simulink library "MBDS_Applications"  (R2018b)
settings: Solver=ode45  StartTime=0.0  StopTime=10.0  RelTol=1e-3
undefined symbols (not defined in the file or in its folder): Ts
libraries: KIBES_Signal x297, simulink x7
(part 3 of 6)

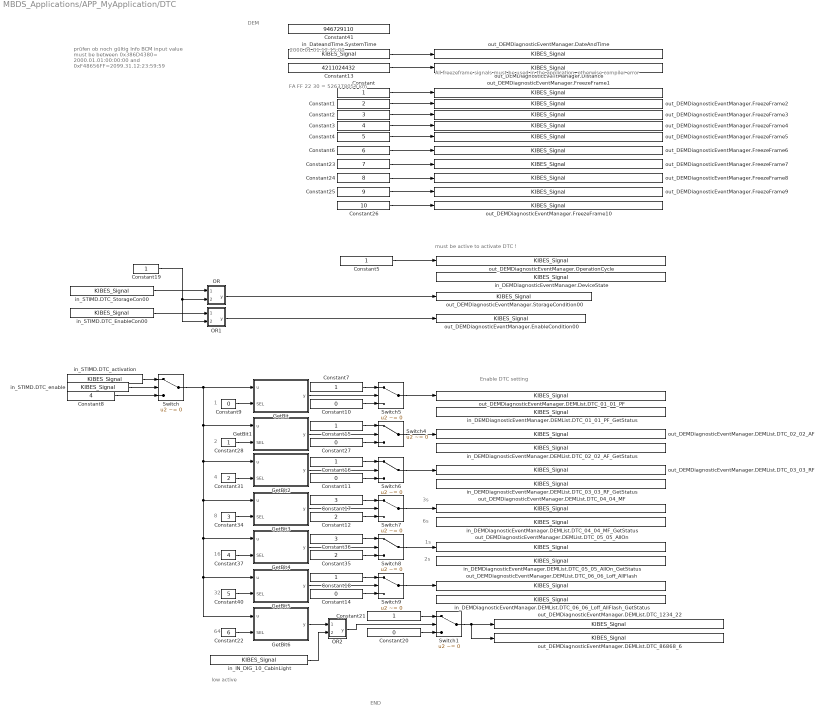
== system MBDS_Applications/APP_MyApplication/DTC ==
  note: 64
  note: FA FF 22 30 = 526378054 km
  note: 2000.01.01:12:15:00
  note: DEM
  note: prüfen ob noch gültig Info BCM
      | input value must be between
      | 0x386D4380= 2000.01.01:00:00:00 and
      | 0xF48656FF=2099.31.12:23:59:59
  note: must be active to activate DTC !
  note: Enable DTC setting
  note: END
  note: 1
  note: 2
  note: 4
  note: 8
  note: 16
  note: 32
  note: 3s
  note: 6s
  note: 1s
  note: 2s
  note: All freezeframe signals must be used in the application, otherwise compiler error
  note: low active
  Constant : Constant  InitFcn=|  OutDataTypeStr=uint16
      | if(exist('MBDS_BlockCallback', 'file'))
      |    MBDS_BlockCallback('Update', gcb);  
      | end
  Constant1 : Constant  InitFcn=|  Value=2  OutDataTypeStr=uint16
      | if(exist('MBDS_BlockCallback', 'file'))
      |    MBDS_BlockCallback('Update', gcb);  
      | end
  Constant10 : Constant  InitFcn=|  Value=0  OutDataTypeStr=uint8
      | if(exist('MBDS_BlockCallback', 'file'))
      |    MBDS_BlockCallback('Update', gcb);  
      | end
  Constant11 : Constant  InitFcn=|  Value=0  OutDataTypeStr=uint8
      | if(exist('MBDS_BlockCallback', 'file'))
      |    MBDS_BlockCallback('Update', gcb);  
      | end
  Constant12 : Constant  InitFcn=|  Value=2  OutDataTypeStr=uint8
      | if(exist('MBDS_BlockCallback', 'file'))
      |    MBDS_BlockCallback('Update', gcb);  
      | end
  Constant13 : Constant  InitFcn=|  Value=4211024432  OutDataTypeStr=uint32
      | if(exist('MBDS_BlockCallback', 'file'))
      |    MBDS_BlockCallback('Update', gcb);  
      | end
  Constant14 : Constant  InitFcn=|  Value=0  OutDataTypeStr=uint8
      | if(exist('MBDS_BlockCallback', 'file'))
      |    MBDS_BlockCallback('Update', gcb);  
      | end
  Constant15 : Constant  InitFcn=|  OutDataTypeStr=uint8
      | if(exist('MBDS_BlockCallback', 'file'))
      |    MBDS_BlockCallback('Update', gcb);  
      | end
  Constant16 : Constant  InitFcn=|  OutDataTypeStr=uint8
      | if(exist('MBDS_BlockCallback', 'file'))
      |    MBDS_BlockCallback('Update', gcb);  
      | end
  Constant17 : Constant  InitFcn=|  Value=3  OutDataTypeStr=uint8
      | if(exist('MBDS_BlockCallback', 'file'))
      |    MBDS_BlockCallback('Update', gcb);  
      | end
  Constant18 : Constant  InitFcn=|  OutDataTypeStr=uint8
      | if(exist('MBDS_BlockCallback', 'file'))
      |    MBDS_BlockCallback('Update', gcb);  
      | end
  Constant19 : Constant  InitFcn=|  OutDataTypeStr=boolean
      | if(exist('MBDS_BlockCallback', 'file'))
      |    MBDS_BlockCallback('Update', gcb);  
      | end
  Constant2 : Constant  InitFcn=|  Value=3  OutDataTypeStr=uint16
      | if(exist('MBDS_BlockCallback', 'file'))
      |    MBDS_BlockCallback('Update', gcb);  
      | end
  Constant20 : Constant  InitFcn=|  Value=0  OutDataTypeStr=uint8
      | if(exist('MBDS_BlockCallback', 'file'))
      |    MBDS_BlockCallback('Update', gcb);  
      | end
  Constant21 : Constant  InitFcn=|  OutDataTypeStr=uint8
      | if(exist('MBDS_BlockCallback', 'file'))
      |    MBDS_BlockCallback('Update', gcb);  
      | end
  Constant22 : Constant  InitFcn=|  Value=6  OutDataTypeStr=uint8
      | if(exist('MBDS_BlockCallback', 'file'))
      |    MBDS_BlockCallback('Update', gcb);  
      | end
  Constant23 : Constant  InitFcn=|  Value=7  OutDataTypeStr=uint16
      | if(exist('MBDS_BlockCallback', 'file'))
      |    MBDS_BlockCallback('Update', gcb);  
      | end
  Constant24 : Constant  InitFcn=|  Value=8  OutDataTypeStr=uint16
      | if(exist('MBDS_BlockCallback', 'file'))
      |    MBDS_BlockCallback('Update', gcb);  
      | end
  Constant25 : Constant  InitFcn=|  Value=9  OutDataTypeStr=uint16
      | if(exist('MBDS_BlockCallback', 'file'))
      |    MBDS_BlockCallback('Update', gcb);  
      | end
  Constant26 : Constant  InitFcn=|  Value=10  OutDataTypeStr=uint16
      | if(exist('MBDS_BlockCallback', 'file'))
      |    MBDS_BlockCallback('Update', gcb);  
      | end
  Constant27 : Constant  InitFcn=|  Value=0  OutDataTypeStr=uint8
      | if(exist('MBDS_BlockCallback', 'file'))
      |    MBDS_BlockCallback('Update', gcb);  
      | end
  Constant28 : Constant  InitFcn=|  OutDataTypeStr=uint8
      | if(exist('MBDS_BlockCallback', 'file'))
      |    MBDS_BlockCallback('Update', gcb);  
      | end
  Constant3 : Constant  InitFcn=|  Value=4  OutDataTypeStr=uint16
      | if(exist('MBDS_BlockCallback', 'file'))
      |    MBDS_BlockCallback('Update', gcb);  
      | end
  Constant31 : Constant  InitFcn=|  Value=2  OutDataTypeStr=uint8
      | if(exist('MBDS_BlockCallback', 'file'))
      |    MBDS_BlockCallback('Update', gcb);  
      | end
  Constant34 : Constant  InitFcn=|  Value=3  OutDataTypeStr=uint8
      | if(exist('MBDS_BlockCallback', 'file'))
      |    MBDS_BlockCallback('Update', gcb);  
      | end
  Constant35 : Constant  InitFcn=|  Value=2  OutDataTypeStr=uint8
      | if(exist('MBDS_BlockCallback', 'file'))
      |    MBDS_BlockCallback('Update', gcb);  
      | end
  Constant36 : Constant  InitFcn=|  Value=3  OutDataTypeStr=uint8
      | if(exist('MBDS_BlockCallback', 'file'))
      |    MBDS_BlockCallback('Update', gcb);  
      | end
  Constant37 : Constant  InitFcn=|  Value=4  OutDataTypeStr=uint8
      | if(exist('MBDS_BlockCallback', 'file'))
      |    MBDS_BlockCallback('Update', gcb);  
      | end
  Constant4 : Constant  InitFcn=|  Value=5  OutDataTypeStr=uint16
      | if(exist('MBDS_BlockCallback', 'file'))
      |    MBDS_BlockCallback('Update', gcb);  
      | end
  Constant40 : Constant  InitFcn=|  Value=5  OutDataTypeStr=uint8
      | if(exist('MBDS_BlockCallback', 'file'))
      |    MBDS_BlockCallback('Update', gcb);  
      | end
  Constant41 : Constant  InitFcn=|  Value=946729110  OutDataTypeStr=uint32
      | if(exist('MBDS_BlockCallback', 'file'))
      |    MBDS_BlockCallback('Update', gcb);  
      | end
  Constant5 : Constant  InitFcn=|  OutDataTypeStr=boolean
      | if(exist('MBDS_BlockCallback', 'file'))
      |    MBDS_BlockCallback('Update', gcb);  
      | end
  Constant6 : Constant  InitFcn=|  Value=6  OutDataTypeStr=uint16
      | if(exist('MBDS_BlockCallback', 'file'))
      |    MBDS_BlockCallback('Update', gcb);  
      | end
  Constant7 : Constant  InitFcn=|  OutDataTypeStr=uint8
      | if(exist('MBDS_BlockCallback', 'file'))
      |    MBDS_BlockCallback('Update', gcb);  
      | end
  Constant8 : Constant  InitFcn=|  Value=4  OutDataTypeStr=uint16
      | if(exist('MBDS_BlockCallback', 'file'))
      |    MBDS_BlockCallback('Update', gcb);  
      | end
  Constant9 : Constant  InitFcn=|  Value=0  OutDataTypeStr=uint8
      | if(exist('MBDS_BlockCallback', 'file'))
      |    MBDS_BlockCallback('Update', gcb);  
      | end
  GetBit : Subsystem  InitFcn=|  mask(GetBit){MBDS_LibraryBlock=on, ZeroIndexing=on, SEL_Enabled=on, SEL=0, MBDS_BlockVersion=08.20.02}
      | if(exist('MBDS_BlockCallback', 'file'))
      |    MBDS_BlockCallback('Update', gcb);
      | end
      mask prompts: MBDS_LibraryBlock "MBDS library block"; ZeroIndexing "Use zero-based indexing"; SEL_Enabled "Show SEL port"; SEL "Bit selection:"; MBDS_BlockVersion "Block version:"
      mask help: Get the value of the specified bit from the input signal.
      mask init: same as MBDS_Applications/APP_MyApplication/NOT
      settings: AttributesFormatString=Zero-based indexing: %<ZeroIndexing>
      mask Help: eval(['open([workdir(''library_dir:''),''\Blockset\help\'',get_param(gcb,''MaskType''),''.html''])'])
      mask Callback ZeroIndexing:
      | % Adopt Value
      | if(exist('MBDS_BlockCallback', 'file'))
      |    MBDS_BlockCallback('ZeroIndexing', gcb);
      | end
      mask Callback SEL_Enabled:
      | % Update mask parameter dialog
      | if(exist('MBDS_BlockCallback', 'file'))
      |    MBDS_BlockCallback('SEL_Enabled', gcb);
      | end
      mask Callback SEL:
      | % Adopt Value
      | if(exist('MBDS_BlockCallback', 'file'))
      |    MBDS_BlockCallback('SEL', gcb);
      | end
      mask DialogControl ParameterTabVar0 Prompt: Main
      mask DialogControl ParameterTabVar01 Prompt: Version
      mask Display:
      | % Show block text
      | disp(sprintf('Get Bit'));
      | 
      | % Display port labels
      | port_label('input', 1, 'u');
      | port_label('input', 2, 'SEL');
      | port_label('output', 1, 'y');
  GetBit1 : Subsystem  InitFcn=|  mask(GetBit){MBDS_LibraryBlock=on, ZeroIndexing=on, SEL_Enabled=on, SEL=0, MBDS_BlockVersion=08.20.02}
      | if(exist('MBDS_BlockCallback', 'file'))
      |    MBDS_BlockCallback('Update', gcb);
      | end
      mask prompts: MBDS_LibraryBlock "MBDS library block"; ZeroIndexing "Use zero-based indexing"; SEL_Enabled "Show SEL port"; SEL "Bit selection:"; MBDS_BlockVersion "Block version:"
      mask help: Get the value of the specified bit from the input signal.
      mask init: same as MBDS_Applications/APP_MyApplication/NOT
      settings: AttributesFormatString=Zero-based indexing: %<ZeroIndexing>
      mask Help: eval(['open([workdir(''library_dir:''),''\Blockset\help\'',get_param(gcb,''MaskType''),''.html''])'])
      mask Callback ZeroIndexing:
      | % Adopt Value
      | if(exist('MBDS_BlockCallback', 'file'))
      |    MBDS_BlockCallback('ZeroIndexing', gcb);
      | end
      mask Callback SEL_Enabled:
      | % Update mask parameter dialog
      | if(exist('MBDS_BlockCallback', 'file'))
      |    MBDS_BlockCallback('SEL_Enabled', gcb);
      | end
      mask Callback SEL:
      | % Adopt Value
      | if(exist('MBDS_BlockCallback', 'file'))
      |    MBDS_BlockCallback('SEL', gcb);
      | end
      mask DialogControl ParameterTabVar0 Prompt: Main
      mask DialogControl ParameterTabVar01 Prompt: Version
      mask Display:
      | % Show block text
      | disp(sprintf('Get Bit'));
      | 
      | % Display port labels
      | port_label('input', 1, 'u');
      | port_label('input', 2, 'SEL');
      | port_label('output', 1, 'y');
  GetBit2 : Subsystem  InitFcn=|  mask(GetBit){MBDS_LibraryBlock=on, ZeroIndexing=on, SEL_Enabled=on, SEL=0, MBDS_BlockVersion=08.20.02}
      | if(exist('MBDS_BlockCallback', 'file'))
      |    MBDS_BlockCallback('Update', gcb);
      | end
      mask prompts: MBDS_LibraryBlock "MBDS library block"; ZeroIndexing "Use zero-based indexing"; SEL_Enabled "Show SEL port"; SEL "Bit selection:"; MBDS_BlockVersion "Block version:"
      mask help: Get the value of the specified bit from the input signal.
      mask init: same as MBDS_Applications/APP_MyApplication/NOT
      settings: AttributesFormatString=Zero-based indexing: %<ZeroIndexing>
      mask Help: eval(['open([workdir(''library_dir:''),''\Blockset\help\'',get_param(gcb,''MaskType''),''.html''])'])
      mask Callback ZeroIndexing:
      | % Adopt Value
      | if(exist('MBDS_BlockCallback', 'file'))
      |    MBDS_BlockCallback('ZeroIndexing', gcb);
      | end
      mask Callback SEL_Enabled:
      | % Update mask parameter dialog
      | if(exist('MBDS_BlockCallback', 'file'))
      |    MBDS_BlockCallback('SEL_Enabled', gcb);
      | end
      mask Callback SEL:
      | % Adopt Value
      | if(exist('MBDS_BlockCallback', 'file'))
      |    MBDS_BlockCallback('SEL', gcb);
      | end
      mask DialogControl ParameterTabVar0 Prompt: Main
      mask DialogControl ParameterTabVar01 Prompt: Version
      mask Display:
      | % Show block text
      | disp(sprintf('Get Bit'));
      | 
      | % Display port labels
      | port_label('input', 1, 'u');
      | port_label('input', 2, 'SEL');
      | port_label('output', 1, 'y');
  GetBit3 : Subsystem  InitFcn=|  mask(GetBit){MBDS_LibraryBlock=on, ZeroIndexing=on, SEL_Enabled=on, SEL=0, MBDS_BlockVersion=08.20.02}
      | if(exist('MBDS_BlockCallback', 'file'))
      |    MBDS_BlockCallback('Update', gcb);
      | end
      mask prompts: MBDS_LibraryBlock "MBDS library block"; ZeroIndexing "Use zero-based indexing"; SEL_Enabled "Show SEL port"; SEL "Bit selection:"; MBDS_BlockVersion "Block version:"
      mask help: Get the value of the specified bit from the input signal.
      mask init: same as MBDS_Applications/APP_MyApplication/NOT
      settings: AttributesFormatString=Zero-based indexing: %<ZeroIndexing>
      mask Help: eval(['open([workdir(''library_dir:''),''\Blockset\help\'',get_param(gcb,''MaskType''),''.html''])'])
      mask Callback ZeroIndexing:
      | % Adopt Value
      | if(exist('MBDS_BlockCallback', 'file'))
      |    MBDS_BlockCallback('ZeroIndexing', gcb);
      | end
      mask Callback SEL_Enabled:
      | % Update mask parameter dialog
      | if(exist('MBDS_BlockCallback', 'file'))
      |    MBDS_BlockCallback('SEL_Enabled', gcb);
      | end
      mask Callback SEL:
      | % Adopt Value
      | if(exist('MBDS_BlockCallback', 'file'))
      |    MBDS_BlockCallback('SEL', gcb);
      | end
      mask DialogControl ParameterTabVar0 Prompt: Main
      mask DialogControl ParameterTabVar01 Prompt: Version
      mask Display:
      | % Show block text
      | disp(sprintf('Get Bit'));
      | 
      | % Display port labels
      | port_label('input', 1, 'u');
      | port_label('input', 2, 'SEL');
      | port_label('output', 1, 'y');
  GetBit4 : Subsystem  InitFcn=|  mask(GetBit){MBDS_LibraryBlock=on, ZeroIndexing=on, SEL_Enabled=on, SEL=0, MBDS_BlockVersion=08.20.02}
      | if(exist('MBDS_BlockCallback', 'file'))
      |    MBDS_BlockCallback('Update', gcb);
      | end
      mask prompts: MBDS_LibraryBlock "MBDS library block"; ZeroIndexing "Use zero-based indexing"; SEL_Enabled "Show SEL port"; SEL "Bit selection:"; MBDS_BlockVersion "Block version:"
      mask help: Get the value of the specified bit from the input signal.
      mask init: same as MBDS_Applications/APP_MyApplication/NOT
      settings: AttributesFormatString=Zero-based indexing: %<ZeroIndexing>
      mask Help: eval(['open([workdir(''library_dir:''),''\Blockset\help\'',get_param(gcb,''MaskType''),''.html''])'])
      mask Callback ZeroIndexing:
      | % Adopt Value
      | if(exist('MBDS_BlockCallback', 'file'))
      |    MBDS_BlockCallback('ZeroIndexing', gcb);
      | end
      mask Callback SEL_Enabled:
      | % Update mask parameter dialog
      | if(exist('MBDS_BlockCallback', 'file'))
      |    MBDS_BlockCallback('SEL_Enabled', gcb);
      | end
      mask Callback SEL:
      | % Adopt Value
      | if(exist('MBDS_BlockCallback', 'file'))
      |    MBDS_BlockCallback('SEL', gcb);
      | end
      mask DialogControl ParameterTabVar0 Prompt: Main
      mask DialogControl ParameterTabVar01 Prompt: Version
      mask Display:
      | % Show block text
      | disp(sprintf('Get Bit'));
      | 
      | % Display port labels
      | port_label('input', 1, 'u');
      | port_label('input', 2, 'SEL');
      | port_label('output', 1, 'y');
  GetBit5 : Subsystem  InitFcn=|  mask(GetBit){MBDS_LibraryBlock=on, ZeroIndexing=on, SEL_Enabled=on, SEL=0, MBDS_BlockVersion=08.20.02}
      | if(exist('MBDS_BlockCallback', 'file'))
      |    MBDS_BlockCallback('Update', gcb);
      | end
      mask prompts: MBDS_LibraryBlock "MBDS library block"; ZeroIndexing "Use zero-based indexing"; SEL_Enabled "Show SEL port"; SEL "Bit selection:"; MBDS_BlockVersion "Block version:"
      mask help: Get the value of the specified bit from the input signal.
      mask init: same as MBDS_Applications/APP_MyApplication/NOT
      settings: AttributesFormatString=Zero-based indexing: %<ZeroIndexing>
      mask Help: eval(['open([workdir(''library_dir:''),''\Blockset\help\'',get_param(gcb,''MaskType''),''.html''])'])
      mask Callback ZeroIndexing:
      | % Adopt Value
      | if(exist('MBDS_BlockCallback', 'file'))
      |    MBDS_BlockCallback('ZeroIndexing', gcb);
      | end
      mask Callback SEL_Enabled:
      | % Update mask parameter dialog
      | if(exist('MBDS_BlockCallback', 'file'))
      |    MBDS_BlockCallback('SEL_Enabled', gcb);
      | end
      mask Callback SEL:
      | % Adopt Value
      | if(exist('MBDS_BlockCallback', 'file'))
      |    MBDS_BlockCallback('SEL', gcb);
      | end
      mask DialogControl ParameterTabVar0 Prompt: Main
      mask DialogControl ParameterTabVar01 Prompt: Version
      mask Display:
      | % Show block text
      | disp(sprintf('Get Bit'));
      | 
      | % Display port labels
      | port_label('input', 1, 'u');
      | port_label('input', 2, 'SEL');
      | port_label('output', 1, 'y');
  GetBit6 : Subsystem  InitFcn=|  mask(GetBit){MBDS_LibraryBlock=on, ZeroIndexing=on, SEL_Enabled=on, SEL=0, MBDS_BlockVersion=08.20.02}
      | if(exist('MBDS_BlockCallback', 'file'))
      |    MBDS_BlockCallback('Update', gcb);
      | end
      mask prompts: MBDS_LibraryBlock "MBDS library block"; ZeroIndexing "Use zero-based indexing"; SEL_Enabled "Show SEL port"; SEL "Bit selection:"; MBDS_BlockVersion "Block version:"
      mask help: Get the value of the specified bit from the input signal.
      mask init: same as MBDS_Applications/APP_MyApplication/NOT
      settings: AttributesFormatString=Zero-based indexing: %<ZeroIndexing>
      mask Help: eval(['open([workdir(''library_dir:''),''\Blockset\help\'',get_param(gcb,''MaskType''),''.html''])'])
      mask Callback ZeroIndexing:
      | % Adopt Value
      | if(exist('MBDS_BlockCallback', 'file'))
      |    MBDS_BlockCallback('ZeroIndexing', gcb);
      | end
      mask Callback SEL_Enabled:
      | % Update mask parameter dialog
      | if(exist('MBDS_BlockCallback', 'file'))
      |    MBDS_BlockCallback('SEL_Enabled', gcb);
      | end
      mask Callback SEL:
      | % Adopt Value
      | if(exist('MBDS_BlockCallback', 'file'))
      |    MBDS_BlockCallback('SEL', gcb);
      | end
      mask DialogControl ParameterTabVar0 Prompt: Main
      mask DialogControl ParameterTabVar01 Prompt: Version
      mask Display:
      | % Show block text
      | disp(sprintf('Get Bit'));
      | 
      | % Display port labels
      | port_label('input', 1, 'u');
      | port_label('input', 2, 'SEL');
      | port_label('output', 1, 'y');
  OR : Subsystem  InitFcn=|  mask(OR){MBDS_LibraryBlock=on, BitwiseMode=off, Inputs=2, UseBitMask=off, BitMask='A1', OutDataTypeStr=Inherit: Inherit via back propagation, MBDS_BlockVersion=07.21.05}
      | if(exist('MBDS_BlockCallback', 'file'))
      |    MBDS_BlockCallback('Update', gcb);
      | end
      mask prompts: MBDS_LibraryBlock "MBDS library block"; BitwiseMode "Use 'bitwise' mode"; Inputs "Number of input ports:"; UseBitMask "Use bit mask"; BitMask "Bit mask:"; OutDataTypeStr "Output data type:"; MBDS_BlockVersion "Version:"
      mask help: Logical or bitwise OR operator. For multiple inputs, operators are applied across the inputs. For a single input, operators are applied across the input vector. In bitwise mode a bit mask can be applied onto single input signals.
      mask init: same as MBDS_Applications/APP_MyApplication/NOT
      mask Help: eval(['open([workdir(''library_dir:''),''\Blockset\help\'',get_param(gcb,''MaskType''),''.html''])'])
      mask Callback BitwiseMode:
      | if(exist('MBDS_BlockCallback', 'file'))
      |    MBDS_BlockCallback('BitwiseMode', gcb);
      | end
      mask Callback Inputs:
      | if(exist('MBDS_BlockCallback', 'file'))
      |    MBDS_BlockCallback('Inputs', gcb);
      | end
      mask Callback UseBitMask:
      | if(exist('MBDS_BlockCallback', 'file'))
      |    MBDS_BlockCallback('UseBitMask', gcb);
      | end
      mask Callback BitMask:
      | if(exist('MBDS_BlockCallback', 'file'))
      |    MBDS_BlockCallback('BitMask', gcb);
      | end
      mask TypeOptions OutDataTypeStr: Inherit: Inherit via back propagation | int8 | uint8 | int16 | uint16 | int32 | uint32 | boolean
      mask Callback OutDataTypeStr:
      | % Adopt Value
      | if(exist('MBDS_BlockCallback', 'file'))
      |    MBDS_BlockCallback('OutDataTypeStr', gcb);
      | end
      mask DialogControl ParameterTabVar0 Prompt: Main
      mask DialogControl ParameterTabVar01 Prompt: Signal Attributes
      mask DialogControl ParameterTabVar012 Prompt: Version
      mask Display:
      | % Show icon or block text
      | if(UseBitMask)
      |    if(isnumeric(BitMask))
      |       BitMaskString = ['0x',dec2hex(floor(BitMask))];
      |    elseif(ischar(BitMask))
      |       BitMaskString = ['0x',upper(BitMask)];
      |    else
      |       BitMaskString = '???';
      |    end
      |    disp(sprintf(['OR\n', BitMaskString]))
      | else
      |    disp('OR')
      | end
  OR1 : Subsystem  InitFcn=|  mask(OR){MBDS_LibraryBlock=on, BitwiseMode=off, Inputs=2, UseBitMask=off, BitMask='A1', OutDataTypeStr=Inherit: Inherit via back propagation, MBDS_BlockVersion=07.21.05}
      | if(exist('MBDS_BlockCallback', 'file'))
      |    MBDS_BlockCallback('Update', gcb);
      | end
      mask prompts: MBDS_LibraryBlock "MBDS library block"; BitwiseMode "Use 'bitwise' mode"; Inputs "Number of input ports:"; UseBitMask "Use bit mask"; BitMask "Bit mask:"; OutDataTypeStr "Output data type:"; MBDS_BlockVersion "Version:"
      mask help: Logical or bitwise OR operator. For multiple inputs, operators are applied across the inputs. For a single input, operators are applied across the input vector. In bitwise mode a bit mask can be applied onto single input signals.
      mask init: same as MBDS_Applications/APP_MyApplication/NOT
      mask Help: eval(['open([workdir(''library_dir:''),''\Blockset\help\'',get_param(gcb,''MaskType''),''.html''])'])
      mask Callback BitwiseMode:
      | if(exist('MBDS_BlockCallback', 'file'))
      |    MBDS_BlockCallback('BitwiseMode', gcb);
      | end
      mask Callback Inputs:
      | if(exist('MBDS_BlockCallback', 'file'))
      |    MBDS_BlockCallback('Inputs', gcb);
      | end
      mask Callback UseBitMask:
      | if(exist('MBDS_BlockCallback', 'file'))
      |    MBDS_BlockCallback('UseBitMask', gcb);
      | end
      mask Callback BitMask:
      | if(exist('MBDS_BlockCallback', 'file'))
      |    MBDS_BlockCallback('BitMask', gcb);
      | end
      mask TypeOptions OutDataTypeStr: Inherit: Inherit via back propagation | int8 | uint8 | int16 | uint16 | int32 | uint32 | boolean
      mask Callback OutDataTypeStr:
      | % Adopt Value
      | if(exist('MBDS_BlockCallback', 'file'))
      |    MBDS_BlockCallback('OutDataTypeStr', gcb);
      | end
      mask DialogControl ParameterTabVar0 Prompt: Main
      mask DialogControl ParameterTabVar01 Prompt: Signal Attributes
      mask DialogControl ParameterTabVar012 Prompt: Version
      mask Display:
      | % Show icon or block text
      | if(UseBitMask)
      |    if(isnumeric(BitMask))
      |       BitMaskString = ['0x',dec2hex(floor(BitMask))];
      |    elseif(ischar(BitMask))
      |       BitMaskString = ['0x',upper(BitMask)];
      |    else
      |       BitMaskString = '???';
      |    end
      |    disp(sprintf(['OR\n', BitMaskString]))
      | else
      |    disp('OR')
      | end
  OR2 : Subsystem  InitFcn=|  mask(OR){MBDS_LibraryBlock=on, BitwiseMode=off, Inputs=2, UseBitMask=off, BitMask='A1', OutDataTypeStr=Inherit: Inherit via back propagation, MBDS_BlockVersion=07.21.05}
      | if(exist('MBDS_BlockCallback', 'file'))
      |    MBDS_BlockCallback('Update', gcb);
      | end
      mask prompts: MBDS_LibraryBlock "MBDS library block"; BitwiseMode "Use 'bitwise' mode"; Inputs "Number of input ports:"; UseBitMask "Use bit mask"; BitMask "Bit mask:"; OutDataTypeStr "Output data type:"; MBDS_BlockVersion "Version:"
      mask help: Logical or bitwise OR operator. For multiple inputs, operators are applied across the inputs. For a single input, operators are applied across the input vector. In bitwise mode a bit mask can be applied onto single input signals.
      mask init: same as MBDS_Applications/APP_MyApplication/NOT
      mask Help: eval(['open([workdir(''library_dir:''),''\Blockset\help\'',get_param(gcb,''MaskType''),''.html''])'])
      mask Callback BitwiseMode:
      | if(exist('MBDS_BlockCallback', 'file'))
      |    MBDS_BlockCallback('BitwiseMode', gcb);
      | end
      mask Callback Inputs:
      | if(exist('MBDS_BlockCallback', 'file'))
      |    MBDS_BlockCallback('Inputs', gcb);
      | end
      mask Callback UseBitMask:
      | if(exist('MBDS_BlockCallback', 'file'))
      |    MBDS_BlockCallback('UseBitMask', gcb);
      | end
      mask Callback BitMask:
      | if(exist('MBDS_BlockCallback', 'file'))
      |    MBDS_BlockCallback('BitMask', gcb);
      | end
      mask TypeOptions OutDataTypeStr: Inherit: Inherit via back propagation | int8 | uint8 | int16 | uint16 | int32 | uint32 | boolean
      mask Callback OutDataTypeStr:
      | % Adopt Value
      | if(exist('MBDS_BlockCallback', 'file'))
      |    MBDS_BlockCallback('OutDataTypeStr', gcb);
      | end
      mask DialogControl ParameterTabVar0 Prompt: Main
      mask DialogControl ParameterTabVar01 Prompt: Signal Attributes
      mask DialogControl ParameterTabVar012 Prompt: Version
      mask Display:
      | % Show icon or block text
      | if(UseBitMask)
      |    if(isnumeric(BitMask))
      |       BitMaskString = ['0x',dec2hex(floor(BitMask))];
      |    elseif(ischar(BitMask))
      |       BitMaskString = ['0x',upper(BitMask)];
      |    else
      |       BitMaskString = '???';
      |    end
      |    disp(sprintf(['OR\n', BitMaskString]))
      | else
      |    disp('OR')
      | end
  Switch : Switch  InitFcn=|  Criteria=u2 ~= 0  OutDataTypeStr=Inherit: Inherit via back propagation  mask(Switch){MBDS_LibraryBlock=on, OutDataTypeStr_=Inherit: Inherit via back propagation, SaturateOnIntegerOverflow_=off, InputSameDT_=off, MBDS_BlockVersion=07.21.05}
      | if(exist('MBDS_BlockCallback', 'file'))
      |    MBDS_BlockCallback('Update', gcb);  
      | end
      mask prompts: MBDS_LibraryBlock "MBDS library block"; OutDataTypeStr_ "Output data type:"; SaturateOnIntegerOverflow_ "Saturate on integer overflow"; InputSameDT_ "Require all inputs to have the same data type"; MBDS_BlockVersion "Block version:"
      mask help: Pass through input 1 when input 2 is not equal to zero; otherwise pass through input 3. The inputs are numbered top to bottom (or left to right). The first and third input ports are data ports, and the second input port is the control port.
      mask init: same as MBDS_Applications/APP_MyApplication/NOT
      mask Help: eval(['open([workdir(''library_dir:''),''\Blockset\help\'',get_param(gcb,''MaskType''),''.html''])'])
      mask TypeOptions OutDataTypeStr_: Inherit: Inherit via back propagation | single | int8 | uint8 | int16 | uint16 | int32 | uint32
      mask DialogControl ParameterTabVar0 Prompt: Signal Attributes
      mask DialogControl ParameterTabVar01 Prompt: Version
  Switch1 : Switch  InitFcn=|  Criteria=u2 ~= 0  OutDataTypeStr=Inherit: Inherit via back propagation  mask(Switch){MBDS_LibraryBlock=on, OutDataTypeStr_=Inherit: Inherit via back propagation, SaturateOnIntegerOverflow_=off, InputSameDT_=off, MBDS_BlockVersion=07.21.05}
      | if(exist('MBDS_BlockCallback', 'file'))
      |    MBDS_BlockCallback('Update', gcb);  
      | end
      mask prompts: MBDS_LibraryBlock "MBDS library block"; OutDataTypeStr_ "Output data type:"; SaturateOnIntegerOverflow_ "Saturate on integer overflow"; InputSameDT_ "Require all inputs to have the same data type"; MBDS_BlockVersion "Block version:"
      mask help: Pass through input 1 when input 2 is not equal to zero; otherwise pass through input 3. The inputs are numbered top to bottom (or left to right). The first and third input ports are data ports, and the second input port is the control port.
      mask init: same as MBDS_Applications/APP_MyApplication/NOT
      mask Help: eval(['open([workdir(''library_dir:''),''\Blockset\help\'',get_param(gcb,''MaskType''),''.html''])'])
      mask TypeOptions OutDataTypeStr_: Inherit: Inherit via back propagation | single | int8 | uint8 | int16 | uint16 | int32 | uint32
      mask DialogControl ParameterTabVar0 Prompt: Signal Attributes
      mask DialogControl ParameterTabVar01 Prompt: Version
  Switch4 : Switch  InitFcn=|  Criteria=u2 ~= 0  OutDataTypeStr=Inherit: Inherit via back propagation  mask(Switch){MBDS_LibraryBlock=on, OutDataTypeStr_=Inherit: Inherit via back propagation, SaturateOnIntegerOverflow_=off, InputSameDT_=off, MBDS_BlockVersion=07.21.05}
      | if(exist('MBDS_BlockCallback', 'file'))
      |    MBDS_BlockCallback('Update', gcb);  
      | end
      mask prompts: MBDS_LibraryBlock "MBDS library block"; OutDataTypeStr_ "Output data type:"; SaturateOnIntegerOverflow_ "Saturate on integer overflow"; InputSameDT_ "Require all inputs to have the same data type"; MBDS_BlockVersion "Block version:"
      mask help: Pass through input 1 when input 2 is not equal to zero; otherwise pass through input 3. The inputs are numbered top to bottom (or left to right). The first and third input ports are data ports, and the second input port is the control port.
      mask init: same as MBDS_Applications/APP_MyApplication/NOT
      mask Help: eval(['open([workdir(''library_dir:''),''\Blockset\help\'',get_param(gcb,''MaskType''),''.html''])'])
      mask TypeOptions OutDataTypeStr_: Inherit: Inherit via back propagation | single | int8 | uint8 | int16 | uint16 | int32 | uint32
      mask DialogControl ParameterTabVar0 Prompt: Signal Attributes
      mask DialogControl ParameterTabVar01 Prompt: Version
  Switch5 : Switch  InitFcn=|  Criteria=u2 ~= 0  OutDataTypeStr=Inherit: Inherit via back propagation  mask(Switch){MBDS_LibraryBlock=on, OutDataTypeStr_=Inherit: Inherit via back propagation, SaturateOnIntegerOverflow_=off, InputSameDT_=off, MBDS_BlockVersion=07.21.05}
      | if(exist('MBDS_BlockCallback', 'file'))
      |    MBDS_BlockCallback('Update', gcb);  
      | end
      mask prompts: MBDS_LibraryBlock "MBDS library block"; OutDataTypeStr_ "Output data type:"; SaturateOnIntegerOverflow_ "Saturate on integer overflow"; InputSameDT_ "Require all inputs to have the same data type"; MBDS_BlockVersion "Block version:"
      mask help: Pass through input 1 when input 2 is not equal to zero; otherwise pass through input 3. The inputs are numbered top to bottom (or left to right). The first and third input ports are data ports, and the second input port is the control port.
      mask init: same as MBDS_Applications/APP_MyApplication/NOT
      mask Help: eval(['open([workdir(''library_dir:''),''\Blockset\help\'',get_param(gcb,''MaskType''),''.html''])'])
      mask TypeOptions OutDataTypeStr_: Inherit: Inherit via back propagation | single | int8 | uint8 | int16 | uint16 | int32 | uint32
      mask DialogControl ParameterTabVar0 Prompt: Signal Attributes
      mask DialogControl ParameterTabVar01 Prompt: Version
  Switch6 : Switch  InitFcn=|  Criteria=u2 ~= 0  OutDataTypeStr=Inherit: Inherit via back propagation  mask(Switch){MBDS_LibraryBlock=on, OutDataTypeStr_=Inherit: Inherit via back propagation, SaturateOnIntegerOverflow_=off, InputSameDT_=off, MBDS_BlockVersion=07.21.05}
      | if(exist('MBDS_BlockCallback', 'file'))
      |    MBDS_BlockCallback('Update', gcb);  
      | end
      mask prompts: MBDS_LibraryBlock "MBDS library block"; OutDataTypeStr_ "Output data type:"; SaturateOnIntegerOverflow_ "Saturate on integer overflow"; InputSameDT_ "Require all inputs to have the same data type"; MBDS_BlockVersion "Block version:"
      mask help: Pass through input 1 when input 2 is not equal to zero; otherwise pass through input 3. The inputs are numbered top to bottom (or left to right). The first and third input ports are data ports, and the second input port is the control port.
      mask init: same as MBDS_Applications/APP_MyApplication/NOT
      mask Help: eval(['open([workdir(''library_dir:''),''\Blockset\help\'',get_param(gcb,''MaskType''),''.html''])'])
      mask TypeOptions OutDataTypeStr_: Inherit: Inherit via back propagation | single | int8 | uint8 | int16 | uint16 | int32 | uint32
      mask DialogControl ParameterTabVar0 Prompt: Signal Attributes
      mask DialogControl ParameterTabVar01 Prompt: Version
  Switch7 : Switch  InitFcn=|  Criteria=u2 ~= 0  OutDataTypeStr=Inherit: Inherit via back propagation  mask(Switch){MBDS_LibraryBlock=on, OutDataTypeStr_=Inherit: Inherit via back propagation, SaturateOnIntegerOverflow_=off, InputSameDT_=off, MBDS_BlockVersion=07.21.05}
      | if(exist('MBDS_BlockCallback', 'file'))
      |    MBDS_BlockCallback('Update', gcb);  
      | end
      mask prompts: MBDS_LibraryBlock "MBDS library block"; OutDataTypeStr_ "Output data type:"; SaturateOnIntegerOverflow_ "Saturate on integer overflow"; InputSameDT_ "Require all inputs to have the same data type"; MBDS_BlockVersion "Block version:"
      mask help: Pass through input 1 when input 2 is not equal to zero; otherwise pass through input 3. The inputs are numbered top to bottom (or left to right). The first and third input ports are data ports, and the second input port is the control port.
      mask init: same as MBDS_Applications/APP_MyApplication/NOT
      mask Help: eval(['open([workdir(''library_dir:''),''\Blockset\help\'',get_param(gcb,''MaskType''),''.html''])'])
      mask TypeOptions OutDataTypeStr_: Inherit: Inherit via back propagation | single | int8 | uint8 | int16 | uint16 | int32 | uint32
      mask DialogControl ParameterTabVar0 Prompt: Signal Attributes
      mask DialogControl ParameterTabVar01 Prompt: Version
  Switch8 : Switch  InitFcn=|  Criteria=u2 ~= 0  OutDataTypeStr=Inherit: Inherit via back propagation  mask(Switch){MBDS_LibraryBlock=on, OutDataTypeStr_=Inherit: Inherit via back propagation, SaturateOnIntegerOverflow_=off, InputSameDT_=off, MBDS_BlockVersion=07.21.05}
      | if(exist('MBDS_BlockCallback', 'file'))
      |    MBDS_BlockCallback('Update', gcb);  
      | end
      mask prompts: MBDS_LibraryBlock "MBDS library block"; OutDataTypeStr_ "Output data type:"; SaturateOnIntegerOverflow_ "Saturate on integer overflow"; InputSameDT_ "Require all inputs to have the same data type"; MBDS_BlockVersion "Block version:"
      mask help: Pass through input 1 when input 2 is not equal to zero; otherwise pass through input 3. The inputs are numbered top to bottom (or left to right). The first and third input ports are data ports, and the second input port is the control port.
      mask init: same as MBDS_Applications/APP_MyApplication/NOT
      mask Help: eval(['open([workdir(''library_dir:''),''\Blockset\help\'',get_param(gcb,''MaskType''),''.html''])'])
      mask TypeOptions OutDataTypeStr_: Inherit: Inherit via back propagation | single | int8 | uint8 | int16 | uint16 | int32 | uint32
      mask DialogControl ParameterTabVar0 Prompt: Signal Attributes
      mask DialogControl ParameterTabVar01 Prompt: Version
  Switch9 : Switch  InitFcn=|  Criteria=u2 ~= 0  OutDataTypeStr=Inherit: Inherit via back propagation  mask(Switch){MBDS_LibraryBlock=on, OutDataTypeStr_=Inherit: Inherit via back propagation, SaturateOnIntegerOverflow_=off, InputSameDT_=off, MBDS_BlockVersion=07.21.05}
      | if(exist('MBDS_BlockCallback', 'file'))
      |    MBDS_BlockCallback('Update', gcb);  
      | end
      mask prompts: MBDS_LibraryBlock "MBDS library block"; OutDataTypeStr_ "Output data type:"; SaturateOnIntegerOverflow_ "Saturate on integer overflow"; InputSameDT_ "Require all inputs to have the same data type"; MBDS_BlockVersion "Block version:"
      mask help: Pass through input 1 when input 2 is not equal to zero; otherwise pass through input 3. The inputs are numbered top to bottom (or left to right). The first and third input ports are data ports, and the second input port is the control port.
      mask init: same as MBDS_Applications/APP_MyApplication/NOT
      mask Help: eval(['open([workdir(''library_dir:''),''\Blockset\help\'',get_param(gcb,''MaskType''),''.html''])'])
      mask TypeOptions OutDataTypeStr_: Inherit: Inherit via back propagation | single | int8 | uint8 | int16 | uint16 | int32 | uint32
      mask DialogControl ParameterTabVar0 Prompt: Signal Attributes
      mask DialogControl ParameterTabVar01 Prompt: Version
  in_DEMDiagnosticEventManager.DEMList.DTC_01_01_PF_GetStatus : KIBES_Signal/KIBES_Signal  MBDS_LibraryBlock=on  DatabaseKey=193  SignalName=DEMDiagnosticEventManager.DEMList.DTC_01_01_PF_GetStatus  SymbolName=DEMDiagnosticEventManager_DEMList_DTC_01_01_PF_GetStatu_000193  DataType=uint8  Init=0  Slope=1  Bias=0  DataSize=1  fpDataType=uint8  BlockIOType=Inport  DeviceType=0
  in_DEMDiagnosticEventManager.DEMList.DTC_02_02_AF_GetStatus : KIBES_Signal/KIBES_Signal  MBDS_LibraryBlock=on  DatabaseKey=194  SignalName=DEMDiagnosticEventManager.DEMList.DTC_02_02_AF_GetStatus  SymbolName=DEMDiagnosticEventManager_DEMList_DTC_02_02_AF_GetStatu_000194  DataType=uint8  Init=0  Slope=1  Bias=0  DataSize=1  fpDataType=uint8  BlockIOType=Inport  DeviceType=0
  in_DEMDiagnosticEventManager.DEMList.DTC_03_03_RF_GetStatus : KIBES_Signal/KIBES_Signal  MBDS_LibraryBlock=on  DatabaseKey=195  SignalName=DEMDiagnosticEventManager.DEMList.DTC_03_03_RF_GetStatus  SymbolName=DEMDiagnosticEventManager_DEMList_DTC_03_03_RF_GetStatu_000195  DataType=uint8  Init=0  Slope=1  Bias=0  DataSize=1  fpDataType=uint8  BlockIOType=Inport  DeviceType=0
  in_DEMDiagnosticEventManager.DEMList.DTC_04_04_MF_GetStatus : KIBES_Signal/KIBES_Signal  MBDS_LibraryBlock=on  DatabaseKey=196  SignalName=DEMDiagnosticEventManager.DEMList.DTC_04_04_MF_GetStatus  SymbolName=DEMDiagnosticEventManager_DEMList_DTC_04_04_MF_GetStatu_000196  DataType=uint8  Init=0  Slope=1  Bias=0  DataSize=1  fpDataType=uint8  BlockIOType=Inport  DeviceType=0
  in_DEMDiagnosticEventManager.DEMList.DTC_05_05_AllOn_GetStatus : KIBES_Signal/KIBES_Signal  MBDS_LibraryBlock=on  DatabaseKey=197  SignalName=DEMDiagnosticEventManager.DEMList.DTC_05_05_AllOn_GetStatus  SymbolName=DEMDiagnosticEventManager_DEMList_DTC_05_05_AllOn_GetSt_000197  DataType=uint8  Init=0  Slope=1  Bias=0  DataSize=1  fpDataType=uint8  BlockIOType=Inport  DeviceType=0
  in_DEMDiagnosticEventManager.DEMList.DTC_06_06_Loff_AllFlash_GetStatus : KIBES_Signal/KIBES_Signal  MBDS_LibraryBlock=on  DatabaseKey=198  SignalName=DEMDiagnosticEventManager.DEMList.DTC_06_06_Loff_AllFlash_GetStatus  SymbolName=DEMDiagnosticEventManager_DEMList_DTC_06_06_Loff_AllFla_000198  DataType=uint8  Init=0  Slope=1  Bias=0  DataSize=1  fpDataType=uint8  BlockIOType=Inport  DeviceType=0
  in_DEMDiagnosticEventManager.DeviceState : KIBES_Signal/KIBES_Signal  MBDS_LibraryBlock=on  DatabaseKey=183  SignalName=DEMDiagnosticEventManager.DeviceState  SymbolName=DEMDiagnosticEventManager_DeviceState_000183  DataType=uint16  Init=0  Slope=1  Bias=0  DataSize=1  fpDataType=uint16  BlockIOType=Inport  DeviceType=0
  in_DateandTime.SystemTime : KIBES_Signal/KIBES_Signal  MBDS_LibraryBlock=on  DatabaseKey=412  SignalName=DateandTime.SystemTime  SymbolName=DateandTime_SystemTime_000412  DataType=uint32  Init=0  Slope=1  Bias=0  DataSize=1  fpDataType=uint32  BlockIOType=Inport  DeviceType=0
  in_IN_DIG_10_CabinLight : KIBES_Signal/KIBES_Signal  MBDS_LibraryBlock=on  DatabaseKey=213  SignalName=IN_DIG_10_CabinLight  SymbolName=IN_DIG_10_CabinLight_000213  DataType=boolean  Init=0  Slope=1  Bias=0  DataSize=1  fpDataType=boolean  BlockIOType=Inport  DeviceType=0
  in_STIMD.DTC_EnableCon00 : KIBES_Signal/KIBES_Signal  MBDS_LibraryBlock=on  DatabaseKey=208  SignalName=STIMD.DTC_EnableCon00  SymbolName=STIMD_DTC_EnableCon00_000208  DataType=boolean  Init=0  Slope=1  Bias=0  DataSize=1  fpDataType=boolean  BlockIOType=Inport  DeviceType=2
  in_STIMD.DTC_StorageCon00 : KIBES_Signal/KIBES_Signal  MBDS_LibraryBlock=on  DatabaseKey=209  SignalName=STIMD.DTC_StorageCon00  SymbolName=STIMD_DTC_StorageCon00_000209  DataType=boolean  Init=0  Slope=1  Bias=0  DataSize=1  fpDataType=boolean  BlockIOType=Inport  DeviceType=2
  in_STIMD.DTC_activation : KIBES_Signal/KIBES_Signal  MBDS_LibraryBlock=on  DatabaseKey=199  SignalName=STIMD.DTC_activation  SymbolName=STIMD_DTC_activation_000199  DataType=uint16  Init=0  Slope=1  Bias=0  DataSize=1  fpDataType=uint16  BlockIOType=Inport  DeviceType=2
  in_STIMD.DTC_enable : KIBES_Signal/KIBES_Signal  MBDS_LibraryBlock=on  DatabaseKey=200  SignalName=STIMD.DTC_enable  SymbolName=STIMD_DTC_enable_000200  DataType=boolean  Init=0  Slope=1  Bias=0  DataSize=1  fpDataType=boolean  BlockIOType=Inport  DeviceType=2
  out_DEMDiagnosticEventManager.DEMList.DTC_01_01_PF : KIBES_Signal/KIBES_Signal  MBDS_LibraryBlock=on  DatabaseKey=192  SignalName=DEMDiagnosticEventManager.DEMList.DTC_01_01_PF  SymbolName=DEMDiagnosticEventManager_DEMList_DTC_01_01_PF_000192  DataType=uint8  Init=0  Slope=1  Bias=0  DataSize=1  fpDataType=uint8  BlockIOType=Outport  DeviceType=0
  out_DEMDiagnosticEventManager.DEMList.DTC_02_02_AF : KIBES_Signal/KIBES_Signal  MBDS_LibraryBlock=on  DatabaseKey=191  SignalName=DEMDiagnosticEventManager.DEMList.DTC_02_02_AF  SymbolName=DEMDiagnosticEventManager_DEMList_DTC_02_02_AF_000191  DataType=uint8  Init=0  Slope=1  Bias=0  DataSize=1  fpDataType=uint8  BlockIOType=Outport  DeviceType=0
  out_DEMDiagnosticEventManager.DEMList.DTC_03_03_RF : KIBES_Signal/KIBES_Signal  MBDS_LibraryBlock=on  DatabaseKey=190  SignalName=DEMDiagnosticEventManager.DEMList.DTC_03_03_RF  SymbolName=DEMDiagnosticEventManager_DEMList_DTC_03_03_RF_000190  DataType=uint8  Init=0  Slope=1  Bias=0  DataSize=1  fpDataType=uint8  BlockIOType=Outport  DeviceType=0
  out_DEMDiagnosticEventManager.DEMList.DTC_04_04_MF : KIBES_Signal/KIBES_Signal  MBDS_LibraryBlock=on  DatabaseKey=189  SignalName=DEMDiagnosticEventManager.DEMList.DTC_04_04_MF  SymbolName=DEMDiagnosticEventManager_DEMList_DTC_04_04_MF_000189  DataType=uint8  Init=0  Slope=1  Bias=0  DataSize=1  fpDataType=uint8  BlockIOType=Outport  DeviceType=0
  out_DEMDiagnosticEventManager.DEMList.DTC_05_05_AllOn : KIBES_Signal/KIBES_Signal  MBDS_LibraryBlock=on  DatabaseKey=188  SignalName=DEMDiagnosticEventManager.DEMList.DTC_05_05_AllOn  SymbolName=DEMDiagnosticEventManager_DEMList_DTC_05_05_AllOn_000188  DataType=uint8  Init=0  Slope=1  Bias=0  DataSize=1  fpDataType=uint8  BlockIOType=Outport  DeviceType=0
  out_DEMDiagnosticEventManager.DEMList.DTC_06_06_Loff_AllFlash : KIBES_Signal/KIBES_Signal  MBDS_LibraryBlock=on  DatabaseKey=187  SignalName=DEMDiagnosticEventManager.DEMList.DTC_06_06_Loff_AllFlash  SymbolName=DEMDiagnosticEventManager_DEMList_DTC_06_06_Loff_AllFla_000187  DataType=uint8  Init=0  Slope=1  Bias=0  DataSize=1  fpDataType=uint8  BlockIOType=Outport  DeviceType=0
  out_DEMDiagnosticEventManager.DEMList.DTC_1234_22 : KIBES_Signal/KIBES_Signal  MBDS_LibraryBlock=on  DatabaseKey=336  SignalName=DEMDiagnosticEventManager.DEMList.DTC_1234_22  SymbolName=DEMDiagnosticEventManager_DEMList_DTC_1234_22_000336  DataType=uint8  Init=0  Slope=1  Bias=0  DataSize=1  fpDataType=uint8  BlockIOType=Outport  DeviceType=0
  out_DEMDiagnosticEventManager.DEMList.DTC_86868_6 : KIBES_Signal/KIBES_Signal  MBDS_LibraryBlock=on  DatabaseKey=337  SignalName=DEMDiagnosticEventManager.DEMList.DTC_86868_6  SymbolName=DEMDiagnosticEventManager_DEMList_DTC_86868_6_000337  DataType=uint8  Init=0  Slope=1  Bias=0  DataSize=1  fpDataType=uint8  BlockIOType=Outport  DeviceType=0
  out_DEMDiagnosticEventManager.DateAndTime : KIBES_Signal/KIBES_Signal  MBDS_LibraryBlock=on  DatabaseKey=182  SignalName=DEMDiagnosticEventManager.DateAndTime  SymbolName=DEMDiagnosticEventManager_DateAndTime_000182  DataType=uint32  Init=0  Slope=1  Bias=0  DataSize=1  fpDataType=uint32  BlockIOType=Outport  DeviceType=0
  out_DEMDiagnosticEventManager.Distance : KIBES_Signal/KIBES_Signal  MBDS_LibraryBlock=on  DatabaseKey=184  SignalName=DEMDiagnosticEventManager.Distance  SymbolName=DEMDiagnosticEventManager_Distance_000184  DataType=uint32  Init=0  Slope=1  Bias=0  DataSize=1  fpDataType=uint32  BlockIOType=Outport  DeviceType=0
  out_DEMDiagnosticEventManager.EnableCondition00 : KIBES_Signal/KIBES_Signal  MBDS_LibraryBlock=on  DatabaseKey=205  SignalName=DEMDiagnosticEventManager.EnableCondition00  SymbolName=DEMDiagnosticEventManager_EnableCondition00_000205  DataType=boolean  Init=0  Slope=1  Bias=0  DataSize=1  fpDataType=boolean  BlockIOType=Outport  DeviceType=0
  out_DEMDiagnosticEventManager.FreezeFrame1 : KIBES_Signal/KIBES_Signal  MBDS_LibraryBlock=on  DatabaseKey=176  SignalName=DEMDiagnosticEventManager.FreezeFrame1  SymbolName=DEMDiagnosticEventManager_FreezeFrame1_000176  DataType=uint16  Init=0  Slope=1  Bias=0  DataSize=1  fpDataType=uint16  BlockIOType=Outport  DeviceType=0
  out_DEMDiagnosticEventManager.FreezeFrame10 : KIBES_Signal/KIBES_Signal  MBDS_LibraryBlock=on  DatabaseKey=409  SignalName=DEMDiagnosticEventManager.FreezeFrame10  SymbolName=DEMDiagnosticEventManager_FreezeFrame10_000409  DataType=uint16  Init=0  Slope=1  Bias=0  DataSize=1  fpDataType=uint16  BlockIOType=Outport  DeviceType=0
  out_DEMDiagnosticEventManager.FreezeFrame2 : KIBES_Signal/KIBES_Signal  MBDS_LibraryBlock=on  DatabaseKey=177  SignalName=DEMDiagnosticEventManager.FreezeFrame2  SymbolName=DEMDiagnosticEventManager_FreezeFrame2_000177  DataType=uint16  Init=0  Slope=1  Bias=0  DataSize=1  fpDataType=uint16  BlockIOType=Outport  DeviceType=0
  out_DEMDiagnosticEventManager.FreezeFrame3 : KIBES_Signal/KIBES_Signal  MBDS_LibraryBlock=on  DatabaseKey=178  SignalName=DEMDiagnosticEventManager.FreezeFrame3  SymbolName=DEMDiagnosticEventManager_FreezeFrame3_000178  DataType=uint16  Init=0  Slope=1  Bias=0  DataSize=1  fpDataType=uint16  BlockIOType=Outport  DeviceType=0
  out_DEMDiagnosticEventManager.FreezeFrame4 : KIBES_Signal/KIBES_Signal  MBDS_LibraryBlock=on  DatabaseKey=179  SignalName=DEMDiagnosticEventManager.FreezeFrame4  SymbolName=DEMDiagnosticEventManager_FreezeFrame4_000179  DataType=uint16  Init=0  Slope=1  Bias=0  DataSize=1  fpDataType=uint16  BlockIOType=Outport  DeviceType=0
  out_DEMDiagnosticEventManager.FreezeFrame5 : KIBES_Signal/KIBES_Signal  MBDS_LibraryBlock=on  DatabaseKey=180  SignalName=DEMDiagnosticEventManager.FreezeFrame5  SymbolName=DEMDiagnosticEventManager_FreezeFrame5_000180  DataType=uint16  Init=0  Slope=1  Bias=0  DataSize=1  fpDataType=uint16  BlockIOType=Outport  DeviceType=0
  out_DEMDiagnosticEventManager.FreezeFrame6 : KIBES_Signal/KIBES_Signal  MBDS_LibraryBlock=on  DatabaseKey=405  SignalName=DEMDiagnosticEventManager.FreezeFrame6  SymbolName=DEMDiagnosticEventManager_FreezeFrame6_000405  DataType=uint16  Init=0  Slope=1  Bias=0  DataSize=1  fpDataType=uint16  BlockIOType=Outport  DeviceType=0
  out_DEMDiagnosticEventManager.FreezeFrame7 : KIBES_Signal/KIBES_Signal  MBDS_LibraryBlock=on  DatabaseKey=406  SignalName=DEMDiagnosticEventManager.FreezeFrame7  SymbolName=DEMDiagnosticEventManager_FreezeFrame7_000406  DataType=uint16  Init=0  Slope=1  Bias=0  DataSize=1  fpDataType=uint16  BlockIOType=Outport  DeviceType=0
  out_DEMDiagnosticEventManager.FreezeFrame8 : KIBES_Signal/KIBES_Signal  MBDS_LibraryBlock=on  DatabaseKey=407  SignalName=DEMDiagnosticEventManager.FreezeFrame8  SymbolName=DEMDiagnosticEventManager_FreezeFrame8_000407  DataType=uint16  Init=0  Slope=1  Bias=0  DataSize=1  fpDataType=uint16  BlockIOType=Outport  DeviceType=0
  out_DEMDiagnosticEventManager.FreezeFrame9 : KIBES_Signal/KIBES_Signal  MBDS_LibraryBlock=on  DatabaseKey=408  SignalName=DEMDiagnosticEventManager.FreezeFrame9  SymbolName=DEMDiagnosticEventManager_FreezeFrame9_000408  DataType=uint16  Init=0  Slope=1  Bias=0  DataSize=1  fpDataType=uint16  BlockIOType=Outport  DeviceType=0
  out_DEMDiagnosticEventManager.OperationCycle : KIBES_Signal/KIBES_Signal  MBDS_LibraryBlock=on  DatabaseKey=181  SignalName=DEMDiagnosticEventManager.OperationCycle  SymbolName=DEMDiagnosticEventManager_OperationCycle_000181  DataType=boolean  Init=0  Slope=1  Bias=0  DataSize=1  fpDataType=boolean  BlockIOType=Outport  DeviceType=0
  out_DEMDiagnosticEventManager.StorageCondition00 : KIBES_Signal/KIBES_Signal  MBDS_LibraryBlock=on  DatabaseKey=206  SignalName=DEMDiagnosticEventManager.StorageCondition00  SymbolName=DEMDiagnosticEventManager_StorageCondition00_000206  DataType=boolean  Init=0  Slope=1  Bias=0  DataSize=1  fpDataType=boolean  BlockIOType=Outport  DeviceType=0
  wires:
  in_DateandTime.SystemTime/1 -> out_DEMDiagnosticEventManager.DateAndTime/1
  in_IN_DIG_10_CabinLight/1 -> OR2/2(u2)
  OR2/1(y) -> Switch1/2
  GetBit6/1(y) -> OR2/1(u1)
  Switch9/1 -> out_DEMDiagnosticEventManager.DEMList.DTC_06_06_Loff_AllFlash/1
  Switch1/1 -> out_DEMDiagnosticEventManager.DEMList.DTC_1234_22/1, out_DEMDiagnosticEventManager.DEMList.DTC_86868_6/1
  Constant26/1 -> out_DEMDiagnosticEventManager.FreezeFrame10/1
  Constant25/1 -> out_DEMDiagnosticEventManager.FreezeFrame9/1
  Constant24/1 -> out_DEMDiagnosticEventManager.FreezeFrame8/1
  Constant23/1 -> out_DEMDiagnosticEventManager.FreezeFrame7/1
  Constant6/1 -> out_DEMDiagnosticEventManager.FreezeFrame6/1
  Constant22/1 -> GetBit6/2(SEL)
  Constant20/1 -> Switch1/3
  Constant21/1 -> Switch1/1
  Switch/1 -> GetBit1/1(u), GetBit2/1(u), GetBit3/1(u), GetBit5/1(u), GetBit6/1(u), GetBit4/1(u), GetBit/1(u)
  Constant19/1 -> OR/2(u2), OR1/2(u2)
  in_STIMD.DTC_EnableCon00/1 -> OR1/1(u1)
  in_STIMD.DTC_StorageCon00/1 -> OR/1(u1)
  OR1/1(y) -> out_DEMDiagnosticEventManager.EnableCondition00/1
  OR/1(y) -> out_DEMDiagnosticEventManager.StorageCondition00/1
  GetBit5/1(y) -> Switch9/2
  GetBit4/1(y) -> Switch8/2
  GetBit3/1(y) -> Switch7/2
  GetBit2/1(y) -> Switch6/2
  Constant40/1 -> GetBit5/2(SEL)
  Constant37/1 -> GetBit4/2(SEL)
  Constant34/1 -> GetBit3/2(SEL)
  Constant31/1 -> GetBit2/2(SEL)
  Constant28/1 -> GetBit1/2(SEL)
  Constant9/1 -> GetBit/2(SEL)
  GetBit/1(y) -> Switch5/2
  in_STIMD.DTC_activation/1 -> Switch/1
  Constant8/1 -> Switch/3
  Switch8/1 -> out_DEMDiagnosticEventManager.DEMList.DTC_05_05_AllOn/1
  Constant14/1 -> Switch9/3
  Constant18/1 -> Switch9/1
  Constant35/1 -> Switch8/3
  Constant36/1 -> Switch8/1
  Constant12/1 -> Switch7/3
  Constant17/1 -> Switch7/1
  Switch7/1 -> out_DEMDiagnosticEventManager.DEMList.DTC_04_04_MF/1
  Constant11/1 -> Switch6/3
  Constant16/1 -> Switch6/1
  Switch6/1 -> out_DEMDiagnosticEventManager.DEMList.DTC_03_03_RF/1
  Constant27/1 -> Switch4/3
  Constant15/1 -> Switch4/1
  Switch4/1 -> out_DEMDiagnosticEventManager.DEMList.DTC_02_02_AF/1
  GetBit1/1(y) -> Switch4/2
  Constant10/1 -> Switch5/3
  Constant7/1 -> Switch5/1
  Switch5/1 -> out_DEMDiagnosticEventManager.DEMList.DTC_01_01_PF/1
  in_STIMD.DTC_enable/1 -> Switch/2
  Constant13/1 -> out_DEMDiagnosticEventManager.Distance/1
  Constant5/1 -> out_DEMDiagnosticEventManager.OperationCycle/1
  Constant4/1 -> out_DEMDiagnosticEventManager.FreezeFrame5/1
  Constant3/1 -> out_DEMDiagnosticEventManager.FreezeFrame4/1
  Constant2/1 -> out_DEMDiagnosticEventManager.FreezeFrame3/1
  Constant1/1 -> out_DEMDiagnosticEventManager.FreezeFrame2/1
  Constant/1 -> out_DEMDiagnosticEventManager.FreezeFrame1/1
